simulink model "cell_model"  (R2020b)
settings: Solver=VariableStepAuto  StartTime=0.0  StopTime=t_end  MaxStep=0.1  RelTol=1e-6
values from neighbouring files (symbols this model uses):
  A_an = 2.5e13    (= 25000000000000)    [main_cell.m]
  A_ca = 2.55e14    (= 255000000000000)    [main_cell.m]
  A_sei = 2.25e15    (= 2.25e+15)    [main_cell.m]
  capacity = 4.5    [Cell_1_RC_25.mat]    (also in Cell_43_RC_25.mat; parameters.mat = 10)
  E_an = 2.24e-19    [main_cell.m]
  E_ca = 2.64e-19    [main_cell.m]
  E_sei = 2.24e-19    [main_cell.m]
  h_an = 1714*1000    (= 1714000)    [main_cell.m]
  h_ca = 790*1000    (= 790000)    [main_cell.m]
  h_sei = 257*1000    (= 257000)    [main_cell.m]
  k_b = 1.3806e-23    [main_cell.m]
  m_an = 19.107/1000    (= 0.019107)    [main_cell.m]
  m_ca = 36.56/1000    (= 0.03656)    [main_cell.m]
  Q = capacity*3600*num_cells    [main.m]    (also in main_1S2P.m; main_cell.m = 4.6)
  SOC_0 = 1    [main.m]    (also in main_1S2P.m; main_cell.m)
  x_an_0 = 0.75    [main_cell.m]
  x_sei_0 = 0.15    [main_cell.m]
  z_0 = 0.033    [main_cell.m]
undefined symbols (not defined in the file or in its folder): Battery, LiBatteryElements_lib, T_init
libraries: fl_lib x20, nesl_utility x15, Copy_of_LiBatteryElements_lib x4, simulink x1
settings Model: Creator=Vivian  LastModifiedBy=Vivian
settings SolverCC: ZeroCrossAlgorithm=Adaptive
settings DebuggingCC: IgnoredZcDiagnostic=none

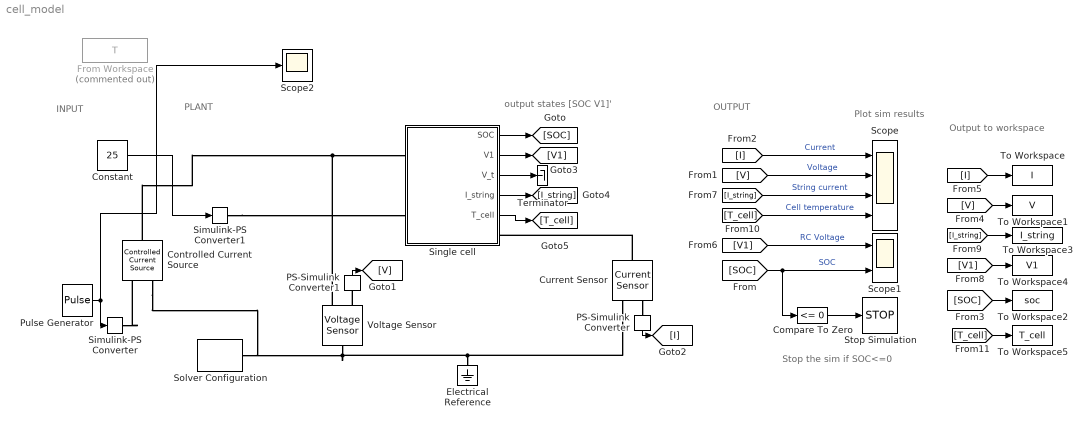
== system cell_model ==
  note: output states [SOC V1]'
  note: Output to workspace
  note: Plot sim results
  note: Stop the sim if SOC<=0
  note: PLANT
  note: INPUT
  note: OUTPUT
  Compare To Zero : simulink/Logic and Bit Operations/Compare To Zero  relop=<=  OutDataTypeStr=boolean
  Constant : Constant  Value=25
  Controlled Current Source : fl_lib/Electrical/Electrical Sources/Controlled Current Source
  Current Sensor : fl_lib/Electrical/Electrical Sensors/Current Sensor
  Electrical Reference : fl_lib/Electrical/Electrical Elements/Electrical Reference
  From Workspace : FromWorkspace  Commented=on  VariableName=T
  PS-Simulink Converter : nesl_utility/PS-Simulink Converter  PhysicalDomain=network_engine_domain  SubClassName=ps_output  LeftPortType=input  RightPortType=output  PseudoPeriodic=off  Frequencies=[]  Unit=inherit  AffineConversion=off
  PS-Simulink Converter1 : nesl_utility/PS-Simulink Converter  PhysicalDomain=network_engine_domain  SubClassName=ps_output  LeftPortType=input  RightPortType=output  PseudoPeriodic=off  Frequencies=[]  Unit=inherit  AffineConversion=off
  Pulse Generator : DiscretePulseGenerator  PulseType=Time based  Amplitude=9  Period=7*60  PulseWidth=2/7*100
  Scope : Scope  NumInputPorts=4
  Scope1 : Scope  NumInputPorts=2
  Scope2 : Scope
  Simulink-PS Converter : nesl_utility/Simulink-PS Converter  PhysicalDomain=network_engine_domain  SubClassName=ps_input  LeftPortType=input  RightPortType=output  PseudoPeriodic=off  Frequencies=[]  NoiseDistribution=none  NoiseParameters=[]  Unit=1  AffineConversion=off  FilteringAndDerivatives=provide  SimscapeFilterOrder=1  InputFilterTimeConstant=0.001  UdotUserProvided=0
  Simulink-PS Converter1 : nesl_utility/Simulink-PS Converter  PhysicalDomain=network_engine_domain  SubClassName=ps_input  LeftPortType=input  RightPortType=output  PseudoPeriodic=off  Frequencies=[]  NoiseDistribution=none  NoiseParameters=[]  Unit=1  AffineConversion=off  FilteringAndDerivatives=provide  SimscapeFilterOrder=1  InputFilterTimeConstant=0.001  UdotUserProvided=0
  Single cell : Subsystem
  Solver Configuration : nesl_utility/Solver Configuration  PhysicalDomain=network_engine_domain  SubClassName=solver  LeftPortType=input  RightPortType=generic  Tones=[]  Harmonics=[]  SimulateNoise=off  Profile=off  UseLocalSampling=off  EnableSwitchedLinearOptims=on  FrequencyDomain=off  UseCCode=off  RelTol=0.001  AbsTol=1e-06  MinStep=1e-09  ToWorkspace=off  RevertToSquareIcSolve=off  NumHomotopyIterations=100  PhasorMode=off  PhasorModeNumHarmonics=1  DoDC=off  ResidualTolerance=1e-09  UseLocalSolver=off  LocalSolverChoice=NE_BACKWARD_EULER_ADVANCER  LocalSolverSampleTime=0.001  DoFixedCost=off  MaxNonlinIter=3  MaxModeIter=2  ComputeImpulses=off  ImpulseIterations=2  LinearAlgebra=auto  EquationFormulation=NE_TIME_EF  DelaysMemoryBudget=1024  AutomaticFiltering=on  FilteringTimeConstant=0.001  PartitionStorageMethod=AS_NEEDED  PartitionMemoryBudget=1024  PartitionMethod=ROBUST
  Stop Simulation : Stop
  Terminator : Terminator
  To Workspace : ToWorkspace  VariableName=I  SampleTime=-1
  To Workspace1 : ToWorkspace  VariableName=V  SampleTime=-1
  To Workspace2 : ToWorkspace  VariableName=soc  SampleTime=-1
  To Workspace3 : ToWorkspace  VariableName=I_string  SampleTime=-1
  To Workspace4 : ToWorkspace  VariableName=V1  SampleTime=-1
  To Workspace5 : ToWorkspace  VariableName=T_cell  SampleTime=-1
  Voltage Sensor : fl_lib/Electrical/Electrical Sensors/Voltage Sensor
  wires:
  Compare To Zero/1 -> Stop Simulation/1
  Single cell/1(SOC) -> [SOC]
  [SOC] -> Compare To Zero/1, Scope1/2  "SOC"
  [V] -> Scope/2  "Voltage"
  PS-Simulink Converter/1 -> [I]
  PS-Simulink Converter1/1 -> [V]
  [I] -> Scope/1  "Current"
  [I] -> To Workspace/1
  [V] -> To Workspace1/1
  [SOC] -> To Workspace2/1
  Constant/1 -> Simulink-PS Converter1/1
  Single cell/3(V_t) -> Terminator/1
  Single cell/2(V1) -> [V1]
  Single cell/4(I_string) -> [I_string]
  [V1] -> To Workspace4/1
  [I_string] -> To Workspace3/1
  [V1] -> Scope1/1  "RC Voltage"
  Single cell/5(T_cell) -> [T_cell]
  [I_string] -> Scope/3  "String current"
  [T_cell] -> Scope/4  "Cell temperature"
  Pulse Generator/1 -> Scope2/1, Simulink-PS Converter/1
  [T_cell] -> To Workspace5/1
  connections:
  Current Sensor/RConn2 -- Electrical Reference/LConn1 -- Controlled Current Source/RConn2 -- Solver Configuration/RConn1 -- Voltage Sensor/LConn1
  Voltage Sensor/RConn1 -- PS-Simulink Converter1/LConn1
  Voltage Sensor/RConn2 -- Controlled Current Source/LConn1 -- Single cell/LConn1
  Current Sensor/LConn1 -- Single cell/RConn1
  Current Sensor/RConn1 -- PS-Simulink Converter/LConn1
  Simulink-PS Converter1/RConn1 -- Single cell/LConn2
  Simulink-PS Converter/RConn1 -- Controlled Current Source/RConn1

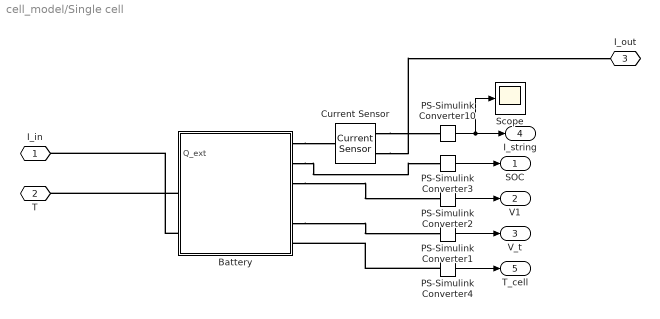
== system cell_model/Single cell ==
  Battery : Subsystem  AncestorBlock=LiBatteryElements_lib/Battery
  Current Sensor : fl_lib/Electrical/Electrical Sensors/Current Sensor
  PS-Simulink Converter{1..4,10} (5 alike) : nesl_utility/PS-Simulink Converter  PhysicalDomain=network_engine_domain  SubClassName=ps_output  LeftPortType=input  RightPortType=output  PseudoPeriodic=off  Frequencies=[]  Unit=inherit  AffineConversion=off
  Scope : Scope
  I_in : PMIOPort  Side=Left
  T : PMIOPort  Port=2  Side=Left
  I_out : PMIOPort  Port=3  Side=Right
  SOC : Outport
  V1 : Outport  Port=2
  V_t : Outport  Port=3
  I_string : Outport  Port=4
  T_cell : Outport  Port=5
  wires:
  PS-Simulink Converter2/1 -> V1/1
  PS-Simulink Converter3/1 -> SOC/1
  PS-Simulink Converter1/1 -> V_t/1
  PS-Simulink Converter10/1 -> Scope/1, I_string/1
  PS-Simulink Converter4/1 -> T_cell/1
  connections:
  Current Sensor/RConn2 -- I_out/RConn1
  Battery/LConn1 -- I_in/RConn1
  Battery/LConn2 -- T/RConn1
  Current Sensor/RConn1 -- PS-Simulink Converter10/LConn1
  Battery/RConn1 -- Current Sensor/LConn1
  PS-Simulink Converter4/LConn1 -- Battery/RConn6
  Battery/RConn5 -- PS-Simulink Converter1/LConn1
  Battery/RConn3 -- PS-Simulink Converter2/LConn1
  Battery/RConn2 -- PS-Simulink Converter3/LConn1

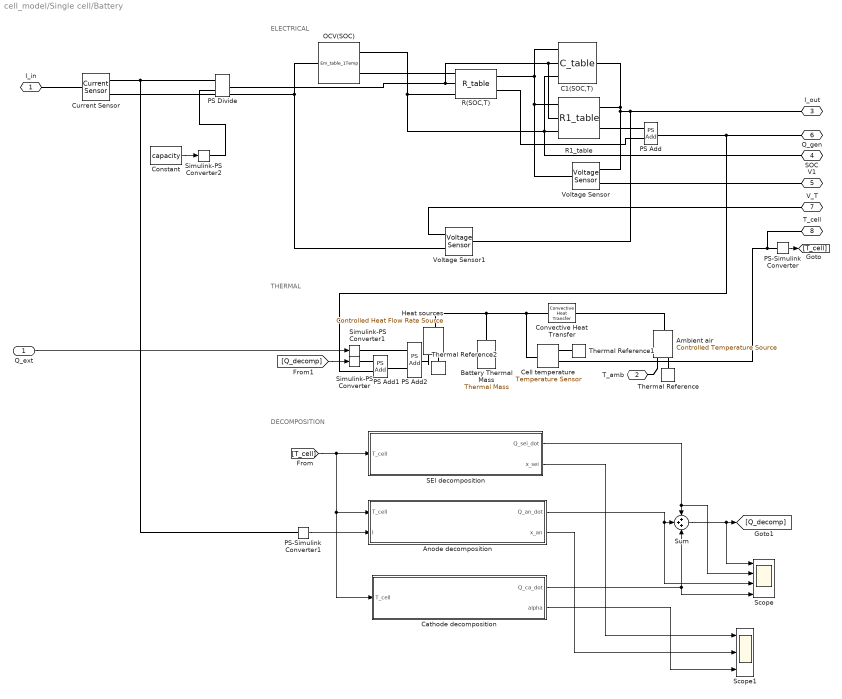
== system cell_model/Single cell/Battery ==
  note: DECOMPOSITION
  note: THERMAL
  note: ELECTRICAL
  Q_ext : Inport
  Ambient air : fl_lib/Thermal/Thermal Sources/Controlled Temperature Source
  Anode decomposition : Subsystem
  Battery Thermal Mass : fl_lib/Thermal/Thermal Elements/Thermal Mass  mass=cell_mass kg  sp_heat=cell_Cp_heat J/kg/K  T_specify=on  T_priority=High  T=T_init K  T_nominal_specify=off  T_nominal_unit=K  T_nominal_value=1  Q_specify=on  Q_priority=None  Q=0 W  Q_nominal_specify=off  Q_nominal_unit=W  Q_nominal_value=1
  C1(SOC,T) : Copy_of_LiBatteryElements_lib/C_table  C_Table=C1 F  SOC_Table=SOC_RC  Temp_Table=T_RC degC  v0=0 V
      settings: InternalSimscapePortConfiguration="{\"Bottom\":[],\"Left\":[{\"id\":\"p\",\"label\":\"+\",\"type\":\"foundation.electrical.electrical\"},{\"id\":\"T\",\"label\":\"T\",\"type\":\"input\"},{\"id\":\"SOC\",\"label\":\"SOC\",\"type\":\"input\"}],\"Right\":[{\"id\":\"n\",\"label\":\"-\",\"type\":\"foundation.electrical.electrical\"}],\"Top\":[]}"
  Cathode decomposition : Subsystem
  Cell temperature : fl_lib/Thermal/Thermal Sensors/Temperature Sensor
  Constant : Constant  Value=capacity
  Convective Heat Transfer : fl_lib/Thermal/Thermal Elements/Convective Heat Transfer  area=cell_area m^2  heat_tr_coeff=h_conv W/(m^2 * K)  T_specify=off  T_priority=None  T=0 K  T_nominal_specify=off  T_nominal_unit=K  T_nominal_value=1  Q_specify=off  Q_priority=None  Q=0 W  Q_nominal_specify=off  Q_nominal_unit=W  Q_nominal_value=1
  Current Sensor : fl_lib/Electrical/Electrical Sensors/Current Sensor
  Heat sources : fl_lib/Thermal/Thermal Sources/Controlled Heat Flow Rate Source
  OCV(SOC) : Copy_of_LiBatteryElements_lib/Em_table_1Temp  Em_Table=OCV V  SOC_Table=SOC_OCV  C=Q hr*A  Qinit=(1-SOC_0)*Q hr*A
      settings: InternalSimscapePortConfiguration="{\"Bottom\":[],\"Left\":[{\"id\":\"p\",\"label\":\"+\",\"type\":\"foundation.electrical.electrical\"},{\"id\":\"SOC\",\"label\":\"SOC\",\"type\":\"output\"}],\"Right\":[{\"id\":\"n\",\"label\":\"-\",\"type\":\"foundation.electrical.electrical\"}],\"Top\":[]}"
  PS Add : fl_lib/Physical Signals/Functions/PS Add
  PS Add1 : fl_lib/Physical Signals/Functions/PS Add
  PS Add2 : fl_lib/Physical Signals/Functions/PS Add
  PS Divide : fl_lib/Physical Signals/Functions/PS Divide
      settings: SourceProductBaseCode=SS
  PS-Simulink Converter : nesl_utility/PS-Simulink Converter  PhysicalDomain=network_engine_domain  SubClassName=ps_output  LeftPortType=input  RightPortType=output  PseudoPeriodic=off  Frequencies=[]  Unit=inherit  AffineConversion=off
  PS-Simulink Converter1 : nesl_utility/PS-Simulink Converter  PhysicalDomain=network_engine_domain  SubClassName=ps_output  LeftPortType=input  RightPortType=output  PseudoPeriodic=off  Frequencies=[]  Unit=inherit  AffineConversion=off
  R(SOC,T) : Copy_of_LiBatteryElements_lib/R_table  R_Table=Rs Ohm  SOC_Table=SOC_RC  Temp_Table=T_RC degC
      settings: InternalSimscapePortConfiguration="{\"Bottom\":[],\"Left\":[{\"id\":\"p\",\"label\":\"+\",\"type\":\"foundation.electrical.electrical\"},{\"id\":\"T\",\"label\":\"T\",\"type\":\"input\"},{\"id\":\"SOC\",\"label\":\"SOC\",\"type\":\"input\"}],\"Right\":[{\"id\":\"n\",\"label\":\"-\",\"type\":\"foundation.electrical.electrical\"},{\"id\":\"pow\",\"label\":\"POW\",\"type\":\"output\"}],\"Top\":[]}"
  R1_table : Copy_of_LiBatteryElements_lib/R1_table  R_Table=R1 Ohm  SOC_Table=SOC_RC  Temp_Table=T_RC K
      settings: InternalSimscapePortConfiguration="{\"Bottom\":[],\"Left\":[{\"id\":\"p\",\"label\":\"+\",\"type\":\"foundation.electrical.electrical\"},{\"id\":\"T\",\"label\":\"T\",\"type\":\"input\"},{\"id\":\"SOC\",\"label\":\"SOC\",\"type\":\"input\"}],\"Right\":[{\"id\":\"n\",\"label\":\"-\",\"type\":\"foundation.electrical.electrical\"},{\"id\":\"pow\",\"label\":\"POW\",\"type\":\"output\"}],\"Top\":[]}"
  SEI decomposition : Subsystem
  Scope : Scope  NumInputPorts=4
  Scope1 : Scope  NumInputPorts=3
  Simulink-PS Converter : nesl_utility/Simulink-PS Converter  PhysicalDomain=network_engine_domain  SubClassName=ps_input  LeftPortType=input  RightPortType=output  PseudoPeriodic=off  Frequencies=[]  NoiseDistribution=none  NoiseParameters=[]  Unit=W  AffineConversion=off  FilteringAndDerivatives=provide  SimscapeFilterOrder=1  InputFilterTimeConstant=0.001  UdotUserProvided=0
  Simulink-PS Converter1 : nesl_utility/Simulink-PS Converter  PhysicalDomain=network_engine_domain  SubClassName=ps_input  LeftPortType=input  RightPortType=output  PseudoPeriodic=off  Frequencies=[]  NoiseDistribution=none  NoiseParameters=[]  Unit=W  AffineConversion=off  FilteringAndDerivatives=provide  SimscapeFilterOrder=1  InputFilterTimeConstant=0.001  UdotUserProvided=0
  Simulink-PS Converter2 : nesl_utility/Simulink-PS Converter  PhysicalDomain=network_engine_domain  SubClassName=ps_input  LeftPortType=input  RightPortType=output  PseudoPeriodic=off  Frequencies=[]  NoiseDistribution=none  NoiseParameters=[]  Unit=1  AffineConversion=off  FilteringAndDerivatives=provide  SimscapeFilterOrder=1  InputFilterTimeConstant=0.001  UdotUserProvided=0
  Sum : Sum  Inputs=+++
  Thermal Reference : fl_lib/Thermal/Thermal Elements/Thermal Reference
  Thermal Reference1 : fl_lib/Thermal/Thermal Elements/Thermal Reference
  Thermal Reference2 : fl_lib/Thermal/Thermal Elements/Thermal Reference
  Voltage Sensor : fl_lib/Electrical/Electrical Sensors/Voltage Sensor
  Voltage Sensor1 : fl_lib/Electrical/Electrical Sensors/Voltage Sensor
  I_in : PMIOPort  Side=Left
  T_amb : PMIOPort  Port=2  Side=Left
  I_out : PMIOPort  Port=3  Side=Right
  SOC : PMIOPort  Port=4  Side=Right
  V1 : PMIOPort  Port=5  Side=Right
  Q_gen : PMIOPort  Port=6  Side=Right
  V_T : PMIOPort  Port=7  Side=Right
  T_cell : PMIOPort  Port=8  Side=Right
  wires:
  PS-Simulink Converter/1 -> [T_cell]
  [Q_decomp] -> Simulink-PS Converter/1
  [T_cell] -> Cathode decomposition/1(T_cell), Anode decomposition/1(T_cell), SEI decomposition/1(T_cell)
  Sum/1 -> Scope/1, [Q_decomp]
  Anode decomposition/1(Q_an_dot) -> Scope/3, Sum/2
  SEI decomposition/1(Q_sei_dot) -> Scope/2, Sum/1
  Cathode decomposition/1(Q_ca_dot) -> Scope/4, Sum/3
  SEI decomposition/2(x_sei) -> Scope1/1
  Anode decomposition/2(x_an) -> Scope1/2
  Cathode decomposition/2(alpha) -> Scope1/3
  Q_ext/1 -> Simulink-PS Converter1/1
  PS-Simulink Converter1/1 -> Anode decomposition/2(I)
  Constant/1 -> Simulink-PS Converter2/1
  connections:
  PS Add/LConn2 -- R(SOC,T)/RConn2
  Voltage Sensor/RConn1 -- V1/RConn1
  Voltage Sensor1/RConn1 -- V_T/RConn1
  PS Add/LConn1 -- R1_table/RConn2
  SOC/RConn1 -- C1(SOC,T)/LConn3 -- R1_table/LConn3 -- OCV(SOC)/LConn2 -- R(SOC,T)/LConn3
  OCV(SOC)/RConn1 -- Voltage Sensor1/RConn2 -- Current Sensor/RConn2
  PS Add/RConn1 -- Q_gen/RConn1 -- PS Add1/LConn2
  R(SOC,T)/LConn1 -- OCV(SOC)/LConn1
  I_out/RConn1 -- Voltage Sensor1/LConn1 -- C1(SOC,T)/RConn1 -- R1_table/RConn1 -- Voltage Sensor/RConn2
  R(SOC,T)/RConn1 -- C1(SOC,T)/LConn1 -- R1_table/LConn1 -- Voltage Sensor/LConn1
  Cell temperature/LConn1 -- Convective Heat Transfer/LConn1 -- Heat sources/LConn1 -- Battery Thermal Mass/LConn1
  Convective Heat Transfer/RConn1 -- Ambient air/LConn1
  Ambient air/RConn1 -- T_amb/RConn1
  Thermal Reference/LConn1 -- Ambient air/RConn2
  Thermal Reference1/LConn1 -- Cell temperature/RConn1
  Thermal Reference2/LConn1 -- Heat sources/RConn2
  PS Add1/LConn1 -- Simulink-PS Converter/RConn1
  PS Add2/LConn2 -- PS Add1/RConn1
  Heat sources/RConn1 -- PS Add2/RConn1
  Simulink-PS Converter1/RConn1 -- PS Add2/LConn1
  Current Sensor/LConn1 -- I_in/RConn1
  Current Sensor/RConn1 -- PS-Simulink Converter1/LConn1 -- PS Divide/LConn1
  Simulink-PS Converter2/RConn1 -- PS Divide/LConn2
  Cell temperature/RConn2 -- T_cell/RConn1 -- PS-Simulink Converter/LConn1
  PS Divide/RConn1 -- R1_table/LConn2 -- C1(SOC,T)/LConn2 -- R(SOC,T)/LConn2

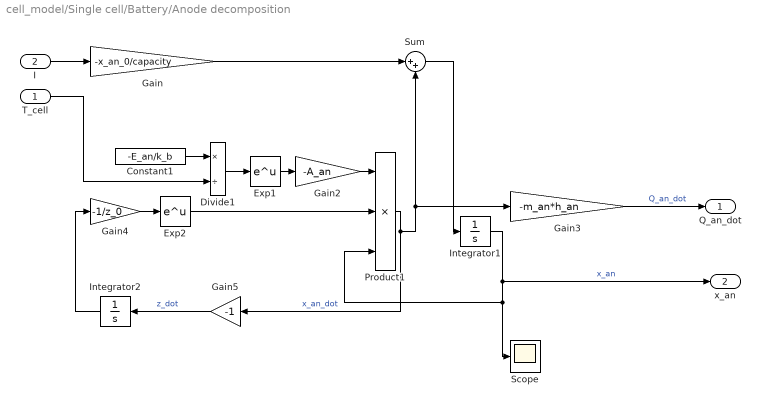
== system cell_model/Single cell/Battery/Anode decomposition ==
  T_cell : Inport
  I : Inport  Port=2
  Constant1 : Constant  Value=-E_an/k_b
  Divide1 : Product  Inputs=*/
  Exp1 : Math  SaturateOnIntegerOverflow=on
  Exp2 : Math  SaturateOnIntegerOverflow=on
  Gain : Gain  Gain=-x_an_0/capacity
  Gain2 : Gain  Gain=-A_an
  Gain3 : Gain  Gain=-m_an*h_an
  Gain4 : Gain  Gain=-1/z_0
  Gain5 : Gain  Gain=-1
  Integrator1 : Integrator  InitialCondition=x_an_0  LimitOutput=on  UpperSaturationLimit=x_an_0  LowerSaturationLimit=0
  Integrator2 : Integrator  InitialCondition=z_0  LimitOutput=on  LowerSaturationLimit=0
  Product1 : Product  Inputs=3
  Scope : Scope
  Sum : Sum  Inputs=|++
  Q_an_dot : Outport
  x_an : Outport  Port=2
  wires:
  Gain2/1 -> Product1/1
  Product1/1 -> Gain5/1, Sum/2, Gain3/1  "x_an_dot"
  Gain5/1 -> Integrator2/1  "z_dot"
  Divide1/1 -> Exp1/1
  Integrator2/1 -> Gain4/1
  Exp1/1 -> Gain2/1
  Integrator1/1 -> Scope/1, Product1/3, x_an/1  "x_an"
  Gain4/1 -> Exp2/1
  Constant1/1 -> Divide1/1
  Exp2/1 -> Product1/2
  Gain3/1 -> Q_an_dot/1  "Q_an_dot"
  T_cell/1 -> Divide1/2
  I/1 -> Gain/1
  Gain/1 -> Sum/1
  Sum/1 -> Integrator1/1

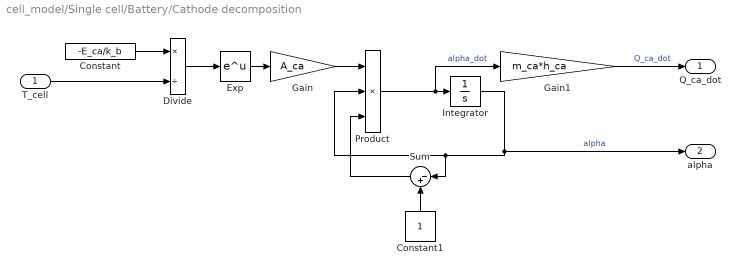
== system cell_model/Single cell/Battery/Cathode decomposition ==
  T_cell : Inport
  Constant : Constant  Value=-E_ca/k_b
  Constant1 : Constant
  Divide : Product  Inputs=*/
  Exp : Math  SaturateOnIntegerOverflow=on
  Gain : Gain  Gain=A_ca
  Gain1 : Gain  Gain=m_ca*h_ca
  Integrator : Integrator  InitialCondition=x_sei_0  LimitOutput=on  UpperSaturationLimit=x_sei_0  LowerSaturationLimit=0
  Product : Product  Inputs=3
  Sum : Sum  Inputs=|-+
  Q_ca_dot : Outport
  alpha : Outport  Port=2
  wires:
  Constant/1 -> Divide/1
  Product/1 -> Gain1/1, Integrator/1  "alpha_dot"
  Gain1/1 -> Q_ca_dot/1  "Q_ca_dot"
  Integrator/1 -> Sum/1, Product/2, alpha/1  "alpha"
  Gain/1 -> Product/1
  T_cell/1 -> Divide/2
  Divide/1 -> Exp/1
  Exp/1 -> Gain/1
  Constant1/1 -> Sum/2
  Sum/1 -> Product/3

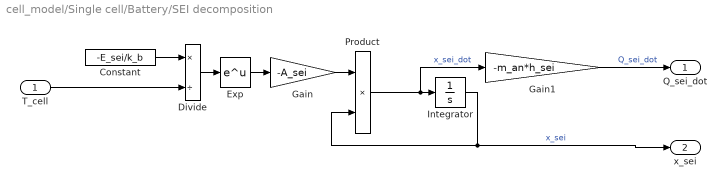
== system cell_model/Single cell/Battery/SEI decomposition ==
  T_cell : Inport
  Constant : Constant  Value=-E_sei/k_b
  Divide : Product  Inputs=*/
  Exp : Math  SaturateOnIntegerOverflow=on
  Gain : Gain  Gain=-A_sei
  Gain1 : Gain  Gain=-m_an*h_sei
  Integrator : Integrator  InitialCondition=x_sei_0  LimitOutput=on  UpperSaturationLimit=x_sei_0  LowerSaturationLimit=0
  Product : Product
  Q_sei_dot : Outport
  x_sei : Outport  Port=2
  wires:
  Constant/1 -> Divide/1
  Product/1 -> Gain1/1, Integrator/1  "x_sei_dot"
  Gain1/1 -> Q_sei_dot/1  "Q_sei_dot"
  Integrator/1 -> x_sei/1, Product/2  "x_sei"
  Gain/1 -> Product/1
  T_cell/1 -> Divide/2
  Divide/1 -> Exp/1
  Exp/1 -> Gain/1
